simulink model "BevDriveCycleBasicModel"  (R2020a)
settings: Solver=VariableStepAuto  StartTime=0.0  StopTime=2474  RelTol=1e-3  AbsTol=1e-3  EnableMultiTasking=on
PreLoadFcn:
  | BevDriveCycleBasicParams
libraries: fl_lib x1, nesl_utility x1
Description:
  | Battery Electric Vehicle drive cycle simulation
settings Model: FPTRunName=Active  Creator=MathWorks  LastModifiedBy=isaacito
settings SolverCC: AutoScaleAbsTol=off
settings DataIOCC: LimitDataPoints=on  MaxDataPoints=15000  SaveFormat=Array  DSMLogging=off
settings OptimizationCC: ExpressionDepthLimit=2147483647  LifeSpan=inf
settings DebuggingCC: UnderspecifiedInitializationDetection=Classic  MergeDetectMultiDrivingBlocksExec=none  FcnCallInpInsideContextMsg=warning  StateNameClashWarn=warning  SFUnexpectedBacktrackingDiag=warning  SFNoUnconditionalDefaultTransitionDiag=warning  SFExecutionAtInitializationDiag=none  ArithmeticOperatorsInVariantConditions=warning
settings HardwareCC: ProdBitPerPointer=32  ProdBitPerSizeT=32  ProdBitPerPtrDiffT=32  ProdLargestAtomicFloat=None  ProdIntDivRoundTo=Undefined  ProdEndianess=Unspecified  ProdWordSize=32  ProdHWDeviceType=32-bit Generic
settings ModelReferenceCC: PropagateSignalLabelsOutOfModel=off
settings SFSimCC: SimUseLocalCustomCode=off  CustomCodeUndefinedFunction=UseInterfaceOnly
settings RTWCC: RTWUseLocalCustomCode=off
settings CodeAppCC: StateflowObjectComments=on
settings GRTTargetCC: TargetLangStandard=C89/C90 (ANSI)  CombineOutputUpdateFcns=off  GRTInterface=on
settings ConfigComp: CovMetricSettings=dw  CovHtmlReporting=on  CovSaveCumulativeToWorkspaceVar=on  CovSaveSingleToWorkspaceVar=on  CovShowResultsExplorer=off  CovExternalEMLEnable=off
settings SimscapeCC: SimscapeLogType=all  SimscapeLogSimulationStatistics=on  SimscapeLogName=logoutssc  SimscapeLogLimitData=off  SimscapeLogDataHistory=10000

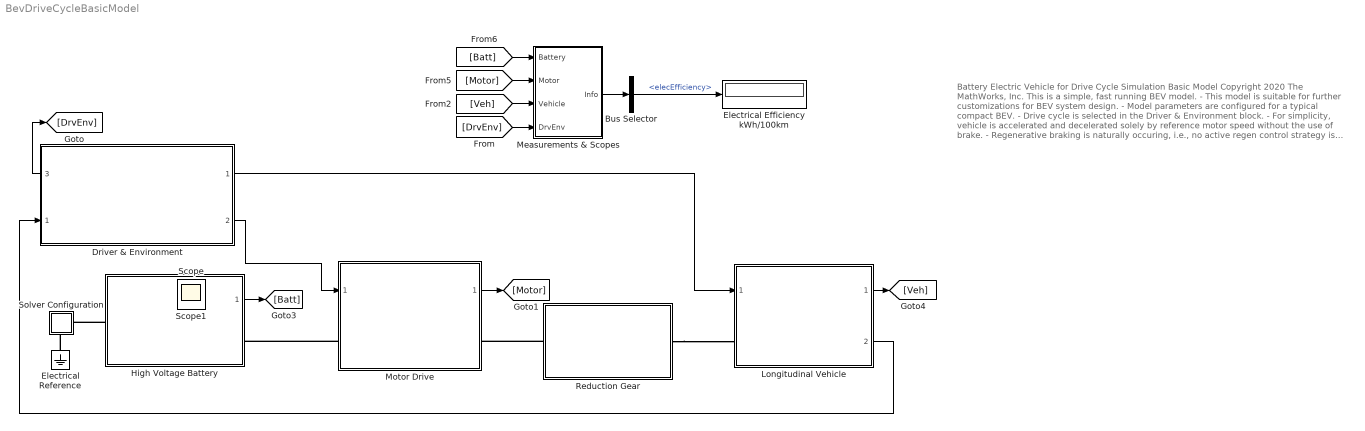
== system BevDriveCycleBasicModel ==
  note: Battery Electric Vehicle for
      | Drive Cycle Simulation
      |
      | Basic Model
      |
      | Copyright 2020 The MathWorks, Inc.
      |
      | This is a simple, fast running BEV model.
      |
      | - This model is suitable for further customizations
      | for BEV system design.
      |
      | - Model parameters are configured for a typical compact BEV.
      |
      | - Drive cycle is selected in the Driver & Environment block.
      |
      | - For simplicity, vehicle is accelerated and decelerated
      | solely by reference motor speed without the use of brake.
      |
      | - Regenerative braking is naturally occuring,
      | i.e., no active regen control strategy is used.
  Bus Selector : BusSelector  OutputSignals=elecEfficiency
  Driver & Environment : Subsystem  ReferencedSubsystem=DirectDriveCycleNoBrakeRefSub
      settings: PortSchema="{\"entries\":[{\"content\":{\"sides\":[{\"content\":{\"connectorIds\":[\"Out3\",\"In1\"]},\"type\":\"ConnectorPlacement.EquallySpacedRectSide\",\"uuid\":\"f589b372-69fb-4153-bcbb-c5cca024a93d\"},{\"content\":{\"connectorIds\":[\"Out1\",\"Out2\"],\"side\":\"RIGHT\"},\"type\":\"ConnectorPlacement.EquallySpacedRectSide\",\"uuid\":\"8e00b759-5def-450b-b0d0-bb2179b3ab27\"},{\"content\":{\"connectorIds\":[],\"side\":\"TOP\"},\"type\":\"ConnectorPlacement.EquallySpacedRectSide\",\"uuid\":\"a456ddaa-2a96-4ebc-8a6c-51aa273a062e\"}]},\"type\":\"ConnectorPlacement.EquallySpacedConnector\",\"uuid\":\"00ab9a78-e98a-4de1-8f67-16ca5fa723c7\"}],\"packageUris\":[\"http://schema.mathworks.com/mf0/Connector/19700101\"],\"version\":\"1.0\"}"
  Electrical Reference : fl_lib/Electrical/Electrical Elements/Electrical Reference
  Electrical Efficiency kWh/100km : Display
  High Voltage Battery : Subsystem  ReferencedSubsystem=BatteryHVBasicRefSub
  Longitudinal Vehicle : Subsystem  ReferencedSubsystem=Vehicle1DBasicRefSub
  Measurements & Scopes : Subsystem
  Motor Drive : Subsystem  ReferencedSubsystem=MotorDriveBasicRefSub
  Reduction Gear : Subsystem  ReferencedSubsystem=ReducerBasicRefSub
  Solver Configuration : Subsystem
      settings: PortSchema="{\"entries\":[{\"content\":{\"sides\":[{\"content\":{\"connectorIds\":[]},\"type\":\"ConnectorPlacement.EquallySpacedRectSide\",\"uuid\":\"4a7e26c2-e9e9-4fea-b605-533b1a682be7\"},{\"content\":{\"connectorIds\":[\"RConn1\"],\"side\":\"RIGHT\"},\"type\":\"ConnectorPlacement.EquallySpacedRectSide\",\"uuid\":\"0210e324-555e-4372-b836-fcc8ab23e933\"},{\"content\":{\"connectorIds\":[],\"side\":\"TOP\"},\"type\":\"ConnectorPlacement.EquallySpacedRectSide\",\"uuid\":\"9bbae011-e6fc-4534-a44f-d79a5697c939\"},{\"content\":{\"connectorIds\":[\"RConn2\"],\"side\":\"BOTTOM\"},\"type\":\"ConnectorPlacement.EquallySpacedRectSide\",\"uuid\":\"d5829c0a-26ea-402d-a1c6-900997ddf1a8\"}]},\"type\":\"ConnectorPlacement.EquallySpacedConnector\",\"uuid\":\"f4e17c65-54c6-42fe-a467-9c6b014b697a\"}],\"packageUris\":[\"http://schema.mathworks.com/mf0/Connector/19700101\"],\"version\":\"1.0\"}"
  Scope : Scope
  Scope1 : Scope
  wires:
  Motor Drive/1 -> [Motor]
  Longitudinal Vehicle/1 -> [Veh]
  [Veh] -> Measurements & Scopes/3(Vehicle)
  [Motor] -> Measurements & Scopes/2(Motor)
  [Batt] -> Measurements & Scopes/1(Battery)
  High Voltage Battery/1 -> [Batt]
  Longitudinal Vehicle/2 -> Driver & Environment/1
  [DrvEnv] -> Measurements & Scopes/4(DrvEnv)
  Measurements & Scopes/1(Info) -> Bus Selector/1
  Bus Selector/1 -> Electrical Efficiency kWh/100km/1  "<elecEfficiency>"
  Driver & Environment/3 -> [DrvEnv]
  Driver & Environment/2 -> Motor Drive/1
  Driver & Environment/1 -> Longitudinal Vehicle/1
  connections:
  Reduction Gear/LConn1 -- Motor Drive/RConn1
  Reduction Gear/RConn1 -- Longitudinal Vehicle/LConn1
  Motor Drive/LConn1 -- High Voltage Battery/RConn1
  High Voltage Battery/LConn1 -- Solver Configuration/RConn1
  Electrical Reference/LConn1 -- Solver Configuration/RConn2

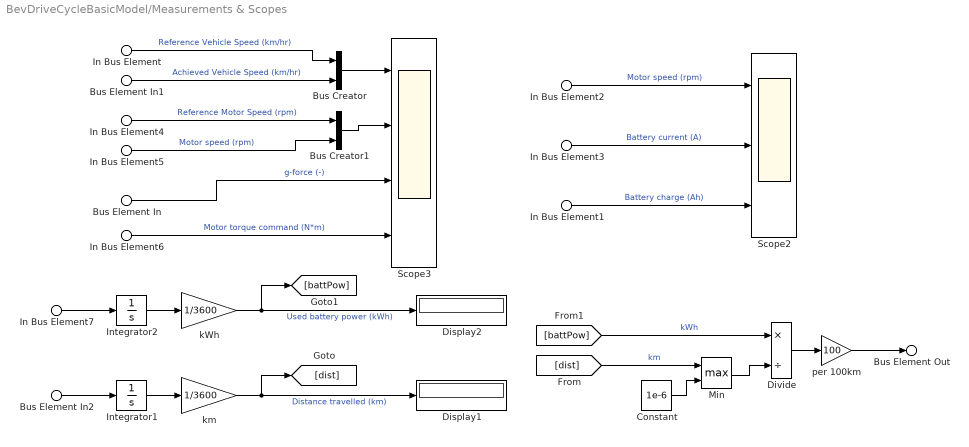
== system BevDriveCycleBasicModel/Measurements & Scopes ==
  In Bus Element3 : Inport  PortName=Battery  Element=Current
  In Bus Element1 : Inport  PortName=Battery  Element=Charge
  In Bus Element7 : Inport  PortName=Battery  Element=Power
      settings: AttributesFormatString=%<Unit>
  In Bus Element6 : Inport  Port=2  PortName=Motor  Element=TrqCmd
      settings: AttributesFormatString=%<Unit>
  In Bus Element5 : Inport  Port=2  PortName=Motor  Element=MotorSpd
      settings: AttributesFormatString=%<Unit>
  In Bus Element2 : Inport  Port=2  PortName=Motor  Element=MotorSpd
      settings: AttributesFormatString=%<Unit>
  Bus Element In : Inport  Port=3  PortName=Vehicle  Element=G
  Bus Element In2 : Inport  Port=3  PortName=Vehicle  Element=VehSpd
      settings: AttributesFormatString=%<Unit>
  Bus Element In1 : Inport  Port=3  PortName=Vehicle  Element=VehSpd
      settings: AttributesFormatString=%<Unit>
  In Bus Element : Inport  Port=4  PortName=DrvEnv  Element=VehSpdRef
  In Bus Element4 : Inport  Port=4  PortName=DrvEnv  Element=MotorSpdRef
  Bus Creator : BusCreator  Inputs=2
  Bus Creator1 : BusCreator  Inputs=2
  Constant : Constant  Value=1e-6
  Display1 : Display
  Display2 : Display
  Divide : Product  Inputs=*/
  Integrator1 : Integrator
  Integrator2 : Integrator
  Min : MinMax  Function=max  Inputs=2
  Scope2 : Scope  NumInputPorts=3
  Scope3 : Scope  NumInputPorts=4
  kWh : Gain  Gain=1/3600
  km : Gain  Gain=1/3600
  per 100km : Gain  Gain=100
  Bus Element Out : Outport  PortName=Info  Element=elecEfficiency
      settings: AttributesFormatString=%<Unit>
  wires:
  In Bus Element1/1 -> Scope2/3  "Battery charge (Ah)"
  In Bus Element3/1 -> Scope2/2  "Battery current (A)"
  Bus Element In2/1 -> Integrator1/1
  Integrator1/1 -> km/1
  km/1 -> [dist], Display1/1  "Distance travelled (km)"
  In Bus Element7/1 -> Integrator2/1
  Integrator2/1 -> kWh/1
  kWh/1 -> [battPow], Display2/1  "Used battery power (kWh)"
  [battPow] -> Divide/1  "kWh"
  Divide/1 -> per 100km/1
  In Bus Element/1 -> Bus Creator/1  "Reference Vehicle Speed (km/hr)"
  Bus Element In1/1 -> Bus Creator/2  "Achieved Vehicle Speed (km/hr)"
  In Bus Element5/1 -> Bus Creator1/2  "Motor speed (rpm)"
  In Bus Element4/1 -> Bus Creator1/1  "Reference Motor Speed (rpm)"
  [dist] -> Min/1  "km"
  Min/1 -> Divide/2
  Constant/1 -> Min/2
  Bus Creator1/1 -> Scope3/2
  In Bus Element2/1 -> Scope2/1  "Motor speed (rpm)"
  per 100km/1 -> Bus Element Out/1
  Bus Element In/1 -> Scope3/3  "g-force (-)"
  Bus Creator/1 -> Scope3/1
  In Bus Element6/1 -> Scope3/4  "Motor torque command (N*m)"

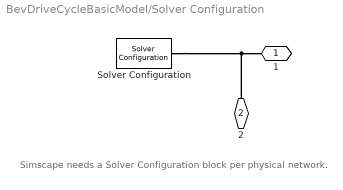
== system BevDriveCycleBasicModel/Solver Configuration ==
  note: Simscape needs a Solver Configuration block per physical network.
  Solver Configuration : nesl_utility/Solver Configuration  PhysicalDomain=network_engine_domain  SubClassName=solver  LeftPortType=input  RightPortType=generic  Tones=[]  Harmonics=[]  SimulateNoise=off  Profile=off  UseLocalSampling=off  EnableSwitchedLinearOptims=on  FrequencyDomain=off  UseCCode=off  RelTol=0.001  AbsTol=1e-06  MinStep=1e-09  ToWorkspace=off  RevertToSquareIcSolve=off  NumHomotopyIterations=100  PhasorMode=off  PhasorModeNumHarmonics=1  DoDC=off  ResidualTolerance=1e-9  UseLocalSolver=off  LocalSolverChoice=NE_BACKWARD_EULER_ADVANCER  LocalSolverSampleTime=0.01  DoFixedCost=off  MaxNonlinIter=3  MaxModeIter=2  LinearAlgebra=auto  EquationFormulation=NE_TIME_EF  DelaysMemoryBudget=1024  AutomaticFiltering=on  FilteringTimeConstant=0.001  PartitionStorageMethod=AS_NEEDED  PartitionMemoryBudget=1024  PartitionMethod=FAST
      settings: AttributesFormatString=Local solver %<UseLocalSolver>
  1 : PMIOPort  Side=Right
  2 : PMIOPort  Port=2  Side=Right
  connections:
  Solver Configuration/RConn1 -- 1/RConn1 -- 2/RConn1
